simulink model "computedTorqueController"  (R2024a)
settings: Solver=ode1  StartTime=0.0  StopTime=10  FixedStep=0.01  RelTol=1e-3
settings Model: Creator=gujun  LastModifiedBy=jun
settings RTWCC: GPUComputeCapability=3.5

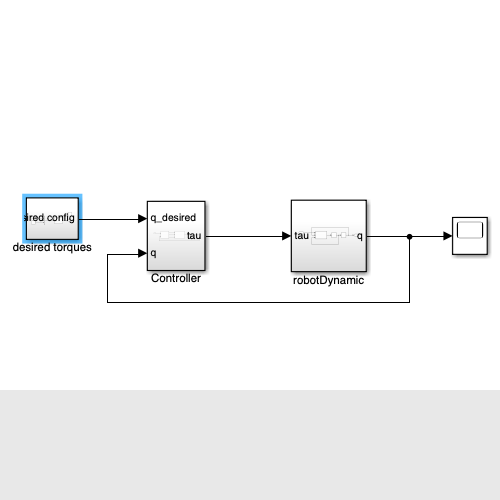
[thumbnail: Simulink's stored preview of the top-level diagram]
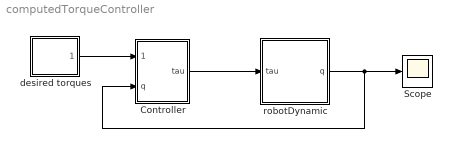
== system computedTorqueController ==
  Controller : Subsystem
  Scope : Scope
  desired torques : Subsystem
  robotDynamic : Subsystem
  wires:
  robotDynamic/1(q) -> Scope/1, Controller/2(q)
  desired torques/1(desired config) -> Controller/1(q_desired)
  Controller/1(tau) -> robotDynamic/1(tau)

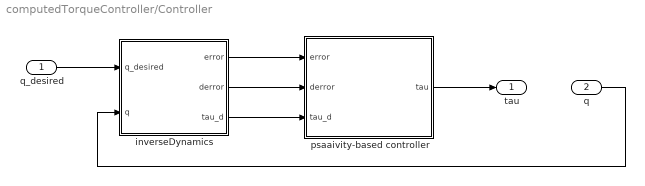
== system computedTorqueController/Controller ==
  q_desired : Inport
  q : Inport  Port=2
  inverseDynamics : Subsystem
  psaaivity-based controller : MATLAB Function  TreatAsAtomicUnit=on
  tau : Outport
  wires:
  q_desired/1 -> inverseDynamics/1(q_desired)
  inverseDynamics/3(tau_d) -> psaaivity-based controller/3(tau_d)
  psaaivity-based controller/1(tau) -> tau/1
  q/1 -> inverseDynamics/2(q)
  inverseDynamics/1(error) -> psaaivity-based controller/1(error)
  inverseDynamics/2(derror) -> psaaivity-based controller/2(derror)

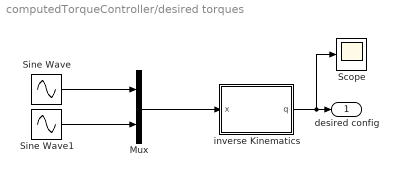
== system computedTorqueController/desired torques ==
  Mux : Mux  Inputs=2
  Scope : Scope
  Sine Wave : Sin  Amplitude=0.2  SampleTime=0
  Sine Wave1 : Sin  Amplitude=0.2  Phase=pi/2  SampleTime=0
  inverse Kinematics : MATLAB Function  TreatAsAtomicUnit=on
  desired config : Outport
  wires:
  Sine Wave1/1 -> Mux/2
  Sine Wave/1 -> Mux/1
  Mux/1 -> inverse Kinematics/1(x)
  inverse Kinematics/1(q) -> Scope/1, desired config/1

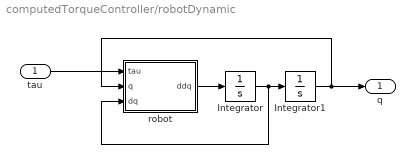
== system computedTorqueController/robotDynamic ==
  tau : Inport
  Integrator : Integrator
  Integrator1 : Integrator
  robot : MATLAB Function  TreatAsAtomicUnit=on
  q : Outport
  wires:
  robot/1(ddq) -> Integrator/1
  tau/1 -> robot/1(tau)
  Integrator1/1 -> q/1, robot/2(q)
  Integrator/1 -> Integrator1/1, robot/3(dq)

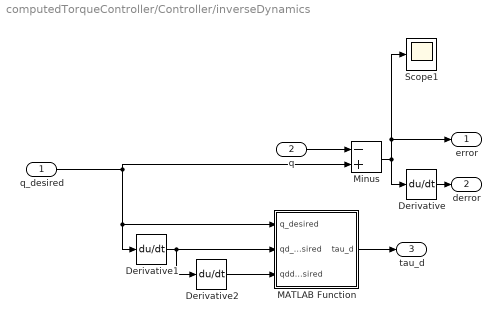
== system computedTorqueController/Controller/inverseDynamics ==
  q_desired : Inport
  q : Inport  Port=2
  Derivative : Derivative
  Derivative1 : Derivative
  Derivative2 : Derivative
  MATLAB Function : MATLAB Function  TreatAsAtomicUnit=on
  Minus : Sum  Inputs=-+
  Scope1 : Scope
  error : Outport
  derror : Outport  Port=2
  tau_d : Outport  Port=3
  wires:
  MATLAB Function/1(tau_d) -> tau_d/1
  Derivative/1 -> derror/1
  q/1 -> Minus/1
  Derivative1/1 -> MATLAB Function/2(qd_desired), Derivative2/1
  q_desired/1 -> Minus/2, MATLAB Function/1(q_desired), Derivative1/1
  Derivative2/1 -> MATLAB Function/3(qdd_desired)
  Minus/1 -> error/1, Scope1/1, Derivative/1

== matlab function computedTorqueController/robotDynamic/robot ==
  data: tau input size=2; ddq output size=2; q input size=2; dq input size=2
function ddq = robot(tau, q, dq)

I1 = 0.05;
m1 = 1.5;
lg1 = 0.2;
lr1 = lg1 / 2;

I2 = 0.01;
m2 = 0.5;
lg2 = 0.2;
lr2 = lg2 / 2;

g = 9.8;

M = [m1 * lr1^2 + I1 + m2 * lg1^2, m2 * lg1 * lr2 * cos(q(2));
        m2 * lg1 * lr2 * cos(q(2)), m2 * lr2^2 + I2];

V = [-m2 * lg1 * lr2 * dq(2)^2 * sin(q(2));
    m2 * lg1 * lr2 * dq(1)^2 * sin(q(2))];

G = [m1 * g * lr1 * cos(q(1)) + m2 * g * lg1 * cos(q(1));
    m2 * g * lr2 * cos(q(1) + q(2));];

ddq = M \ (tau - V - G);

end

== matlab function computedTorqueController/Controller/psaaivity-based controller ==
  data: error input; tau output; derror input; tau_d input
function tau = controller(error, derror, tau_d)

kp = [10, 0;
       0, 10];


kd = [1, 0;
        0, 1];

tau = kp * error + kd * derror + tau_d;

== matlab function computedTorqueController/Controller/inverseDynamics/MATLAB Function ==
  data: tau_d output; q_desired input; qd_desired input; qdd_desired input
function tau_d = dynamics(q_desired, qd_desired, qdd_desired)

I1 = 0.05;
m1 = 1.5;
lg1 = 0.2;
lr1 = lg1 / 2;

I2 = 0.01;
m2 = 0.5;
lg2 = 0.2;
lr2 = lg2 / 2;

g = 9.8;

M = [m1 * lr1^2 + I1 + m2 * lg1^2, m2 * lg1 * lr2 * cos(q_desired(2));
        m2 * lg1 * lr2 * cos(q_desired(2)), m2 * lr2^2 + I2];

V = [-m2 * lg1 * lr2 * qd_desired(2)^2 * sin(q_desired(2));
    m2 * lg1 * lr2 * qd_desired(1)^2 * sin(q_desired(2))];

G = [m1 * g * lr1 * cos(q_desired(1)) + m2 * g * lg1 * cos(q_desired(1));
    m2 * g * lr2 * cos(q_desired(1) + q_desired(2));];

tau_d = M * qdd_desired + V + G;

end

== matlab function computedTorqueController/desired torques/inverse Kinematics ==
  data: x input; q output
function q = inverseKinematics(x)

l1 = 0.2;
l2 = 0.2;


theta_2 = acos((x(1)^2 + x(2)^2 - l1^2 - l2^2) / (2 * l1 * l2));

k1 = l1 + l2 * cos(theta_2);
k2 = l2 * sin(theta_2);

theta_1 = atan2(x(2), x(1)) - atan2(k2, k1);

q = [theta_1;
    theta_2];

end
